simulink model "MassSpringDamper"  (R2025a)
settings: Solver=FixedStepAuto  StartTime=0.0  StopTime=100  FixedStep=0.001  RelTol=1e-3
values from neighbouring files (symbols this model uses):
  b = 0.0458417    [Parameters.m]
  k = 31.17    [Parameters.m]
  m = 0.3027    [Parameters.m]
settings Model: Creator=Yhommy's Notebook  LastModifiedBy=Yhommy's Notebook

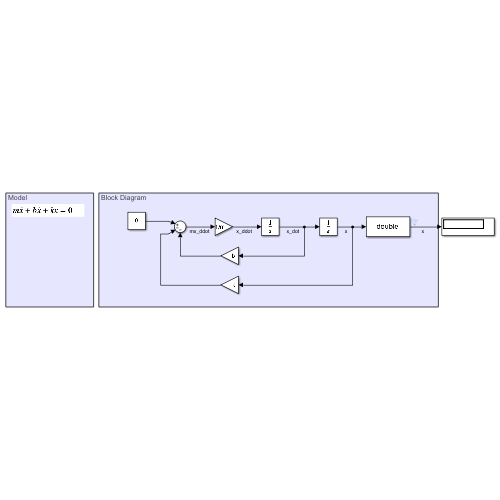
[thumbnail: Simulink's stored preview of the top-level diagram]
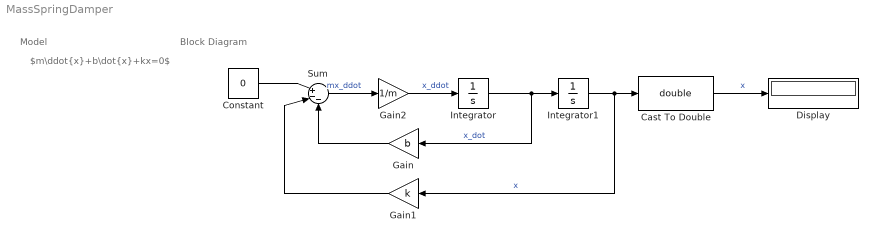
== system MassSpringDamper ==
  note: Block Diagram
  note: $m\ddot{x}+b\dot{x}+kx=0$
  note: Model
  Cast To Double : DataTypeConversion  OutDataTypeStr=double  SaturateOnIntegerOverflow=off  RndMeth=Floor
  Constant : Constant  Value=0
  Display : Display
  Gain : Gain  Gain=b
  Gain1 : Gain  Gain=k
  Gain2 : Gain  Gain=1/m
  Integrator : Integrator
  Integrator1 : Integrator  InitialCondition=-0.08
  Sum : Sum  Inputs=|+--
  wires:
  Integrator/1 -> Gain/1, Integrator1/1  "x_dot"
  Integrator1/1 -> Gain1/1, Cast To Double/1  "x"
  Gain2/1 -> Integrator/1  "x_ddot"
  Sum/1 -> Gain2/1  "mx_ddot"
  Gain/1 -> Sum/3
  Gain1/1 -> Sum/2
  Constant/1 -> Sum/1
  Cast To Double/1 -> Display/1  "x"
